simulink model "Pipe_m_to_m_test"  (R2014b)
settings: Solver=ode23tb  StartTime=0.0  StopTime=10.0  RelTol=1e-3
libraries: DAEMOT_Lib x3
settings Model: Creator=pangbor2  LastModifiedBy=pangbor2

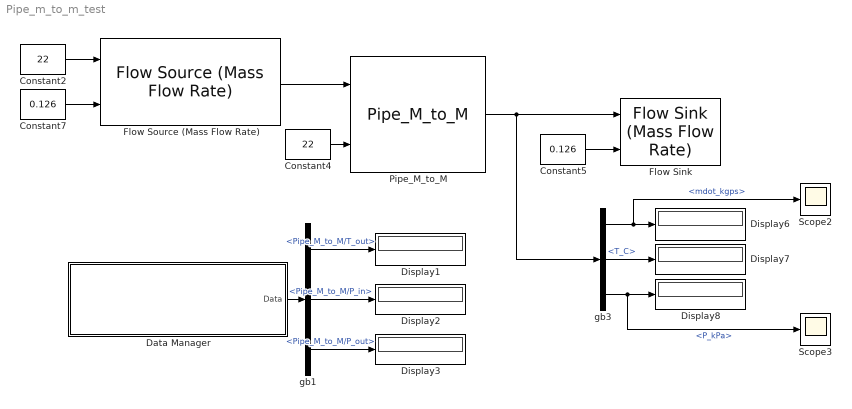
== system Pipe_m_to_m_test ==
  Constant2 : Constant  Value=22
  Constant4 : Constant  Value=22
  Constant5 : Constant  Value=0.126
  Constant7 : Constant  Value=0.126
  Data Manager : Subsystem  AncestorBlock=DAEMOT_Lib/Support Functions/Data Manager  mask{null=0}
      mask init:
      | set_param(gcb, 'LinkStatus', 'inactive')    % disable the library link
      settings: OpenFcn=data_manager
      mask Display: str ='Pipe_M_to_M/T_out\nPipe_M_to_M/P_in\nPipe_M_to_M/P_out'; fprintf(str)
  Display{1..3,6..8} (6 alike) : Display
  Flow Sink : DAEMOT_Lib/Components/Flow Sink (Mass Flow Rate)  M_ext=on  M=0  T_ext=on  T=0  P_ext=on  P=0
  Flow Source (Mass Flow Rate) : DAEMOT_Lib/Components/Flow Source (Mass Flow Rate)  M_ext=on  M=0  T_ext=on  T=0  P_ext=on  P=0
  Pipe_M_to_M : DAEMOT_Lib/Components/Pipe_M_to_M  fld=Water  Tout_init=22  P_init=145  Tamb_init=22  H=0  D=13*1e-3  L=0.2  e=0.01*1e-3
  Scope2 : Scope
      settings: SaveName=ScopeData2
  Scope3 : Scope
      settings: SaveName=ScopeData3
  gb1 : BusSelector  OutputSignals=Pipe_M_to_M/T_out,Pipe_M_to_M/P_in,Pipe_M_to_M/P_out
  gb3 : BusSelector  OutputSignals=mdot_kgps,T_C,P_kPa
  wires:
  Constant7/1 -> Flow Source (Mass Flow Rate)/2
  Constant2/1 -> Flow Source (Mass Flow Rate)/1
  Flow Source (Mass Flow Rate)/1 -> Pipe_M_to_M/1
  Constant5/1 -> Flow Sink/2
  gb3/2 -> Display7/1  "<T_C>"
  gb3/1 -> Scope2/1, Display6/1  "<mdot_kgps>"
  Pipe_M_to_M/1 -> gb3/1, Flow Sink/1
  gb3/3 -> Scope3/1, Display8/1  "<P_kPa>"
  Constant4/1 -> Pipe_M_to_M/2
  Data Manager/1(Data) -> gb1/1
  gb1/1 -> Display1/1  "<Pipe_M_to_M/T_out>"
  gb1/2 -> Display2/1  "<Pipe_M_to_M/P_in>"
  gb1/3 -> Display3/1  "<Pipe_M_to_M/P_out>"

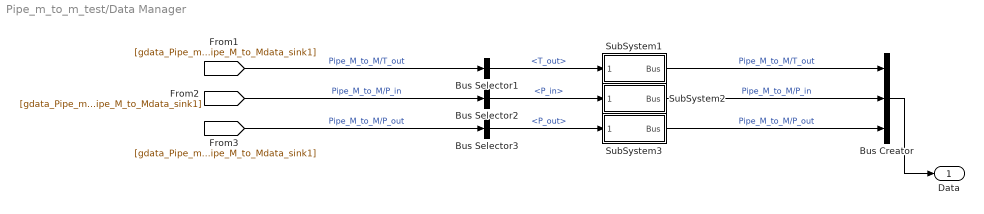
== system Pipe_m_to_m_test/Data Manager ==
  Bus Creator : BusCreator  Inputs=3
  Bus Selector1 : BusSelector  OutputSignals=T_out
  Bus Selector2 : BusSelector  OutputSignals=P_in
  Bus Selector3 : BusSelector  OutputSignals=P_out
  SubSystem1 : Subsystem
  SubSystem2 : Subsystem
  SubSystem3 : Subsystem
  Data : Outport
  wires:
  Bus Creator/1 -> Data/1
  [gdata_Pipe_m_to_m_testPipe_M_to_Mdata_sink1] -> Bus Selector1/1  "Pipe_M_to_M/T_out"
  Bus Selector1/1 -> SubSystem1/1(Rename)  "<T_out>"
  SubSystem1/1(Bus) -> Bus Creator/1  "Pipe_M_to_M/T_out"
  [gdata_Pipe_m_to_m_testPipe_M_to_Mdata_sink1] -> Bus Selector2/1  "Pipe_M_to_M/P_in"
  Bus Selector2/1 -> SubSystem2/1(Rename)  "<P_in>"
  SubSystem2/1(Bus) -> Bus Creator/2  "Pipe_M_to_M/P_in"
  [gdata_Pipe_m_to_m_testPipe_M_to_Mdata_sink1] -> Bus Selector3/1  "Pipe_M_to_M/P_out"
  Bus Selector3/1 -> SubSystem3/1(Rename)  "<P_out>"
  SubSystem3/1(Bus) -> Bus Creator/3  "Pipe_M_to_M/P_out"

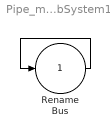
== system Pipe_m_to_m_test/Data Manager/SubSystem1 ==
  Rename : Inport
  Bus : Outport
  wires:
  Rename/1 -> Bus/1

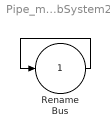
== system Pipe_m_to_m_test/Data Manager/SubSystem2 ==
  Rename : Inport
  Bus : Outport
  wires:
  Rename/1 -> Bus/1

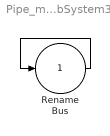
== system Pipe_m_to_m_test/Data Manager/SubSystem3 ==
  Rename : Inport
  Bus : Outport
  wires:
  Rename/1 -> Bus/1
